simulink model "Controlled_full_wave_AC_DC_Wave_SEDC_motor_model"  (R2018a)
settings: Solver=VariableStepAuto  StartTime=0.0  StopTime=0.04  FixedStep=10e-3  MaxStep=10e-3  RelTol=1e-3
values from neighbouring files (symbols this model uses):
  B = 0.01    [AC_DC_Wave_DC_motor_parameters.m]
  J = 5    [AC_DC_Wave_DC_motor_parameters.m]
  K_phi = 1.6    [AC_DC_Wave_DC_motor_parameters.m]
  L = 0.1    [AC_DC_Wave_DC_motor_parameters.m]
  Ra = 0.5    [AC_DC_Wave_DC_motor_parameters.m]
  T_l = 10    [AC_DC_Wave_DC_motor_parameters.m]
libraries: powerlib x12, simulink x2, dspswit3 x1
settings Model: Creator=dell  LastModifiedBy=dell

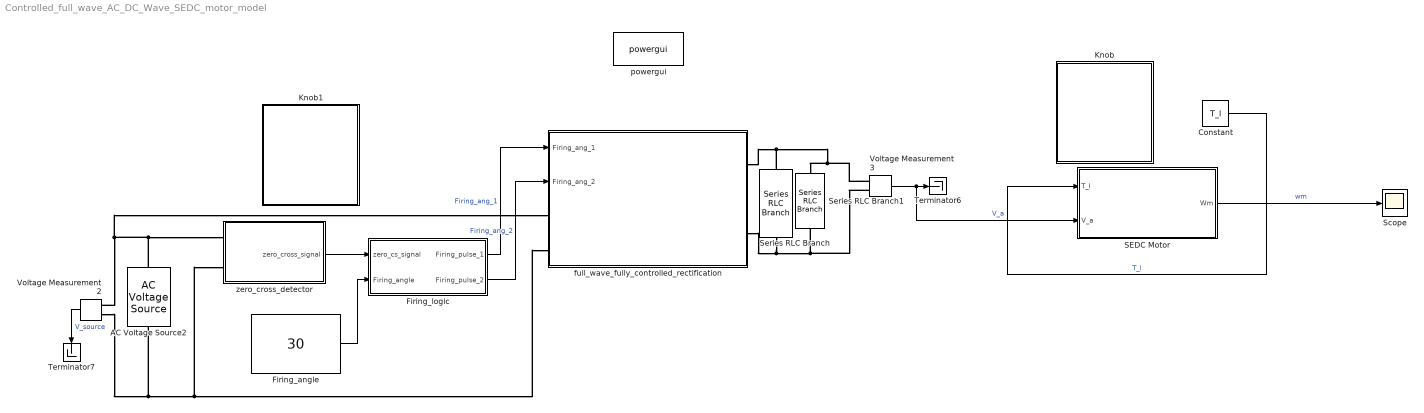
== system Controlled_full_wave_AC_DC_Wave_SEDC_motor_model ==
  AC Voltage Source2 : powerlib/Electrical Sources/AC Voltage Source  Amplitude=sqrt(2)*220  Phase=0  Frequency=50  SampleTime=0  Measurements=None  BusType=swing  Pref=10e3  Qref=0  Qmin=-inf  Qmax=+inf
  Constant : Constant  Value=T_l
  Firing_angle : Constant  Value=30
  Firing_logic : Subsystem
  Knob : Subsystem  DialogController=hmiCreateDDGDialog  IsWebBlock=on  mask(MWDashboardBlock){webBlockId=27bb38d2-9cd0-4bde-b8da-2d6c9efb7173, webBlockType=continuousknob, ShowInLibBrowser=on, ShowInitialText=on, HMISrcModelName=Controlled_full_wave_AC_DC_Wave_SEDC_motor_model}
      mask prompts: webBlockId "WebBlock Id"; webBlockType "WebBlock Type"; HMISrcModelName "Source Model"
      mask help: SimulinkHMI:dialogs:ContinuousKnobDialogDesc
      mask Help: helpview([docroot '/mapfiles/simulink.map'], 'hmi_knob')
      mask Display:
      | if strcmp(get_param(bdroot(gcb),'BlockDiagramType'), 'library')
      |     image([(matlabroot) '/toolbox/simulink/hmi/icons/ContinuousKnob.png']);
      | end
  Knob1 : Subsystem  DialogController=hmiCreateDDGDialog  IsWebBlock=on  mask(MWDashboardBlock){webBlockId=f64e203f-17e4-4edd-b46c-2720ed8f6d71, webBlockType=continuousknob, ShowInLibBrowser=on, ShowInitialText=on, HMISrcModelName=Controlled_full_wave_AC_DC_Wave_SEDC_motor_model}
      mask prompts: webBlockId "WebBlock Id"; webBlockType "WebBlock Type"; HMISrcModelName "Source Model"
      mask help: SimulinkHMI:dialogs:ContinuousKnobDialogDesc
      mask Help: helpview([docroot '/mapfiles/simulink.map'], 'hmi_knob')
      mask Display:
      | if strcmp(get_param(bdroot(gcb),'BlockDiagramType'), 'library')
      |     image([(matlabroot) '/toolbox/simulink/hmi/icons/ContinuousKnob.png']);
      | end
  SEDC Motor : Subsystem  mask{L=L, Ra=Ra, B=B, K_phi=K_phi, J=J}
      mask prompts: L "Inductance"; Ra "Resistance"; B "Damping"; K_phi "Motor Constant"; J "Inertia"
  Scope : Scope
  Series RLC Branch : powerlib/Elements/Series RLC Branch  LConnTagsString=__new0  RConnTagsString=__new0  BranchType=C  Resistance=1  Inductance=1e-3  SetiL0=off  InitialCurrent=0  Capacitance=1  Setx0=off  InitialVoltage=0  Measurements=None
  Series RLC Branch1 : powerlib/Elements/Series RLC Branch  LConnTagsString=__new0  RConnTagsString=__new0  BranchType=R  Resistance=50  Inductance=1e-3  SetiL0=off  InitialCurrent=0  Capacitance=1e-6  Setx0=off  InitialVoltage=0  Measurements=None
  Terminator6 : Terminator
  Terminator7 : Terminator
  Voltage Measurement2 : powerlib/Measurements/Voltage Measurement  PhasorSimulation=off  OutputType=Complex  PSBequivalent=0
  Voltage Measurement3 : powerlib/Measurements/Voltage Measurement  PhasorSimulation=off  OutputType=Complex  PSBequivalent=0
  full_wave_fully_controlled_rectification : Subsystem
  powergui : powerlib/powergui  Priority=1  SimulationMode=Discrete  SampleTime=50e-6  frequency=60  Iterations=50  frequencyindice=0  Pbase=100e6  ErrMax=1e-4  UnitsV=kV  UnitsW=MW  buscounter=0  FunctionMessages=off  echomessages=off  EnableUseOfTLC=off  CurrentSourceSwitches=off  DisableSnubberDevices=off  DisableRonSwitches=off  DisableVfSwitches=off  DisplayEquations=off  SolverType=Tustin/Backward Euler (TBE)  Interpol=off  ExternalGateDelay=off  methode=off  Ts=100  x0status=blocks  SPID=off  SwTol=0  HookPort=off  RestoreLinks=warning  ResistiveCurrentMeasurement=off  Frange=[0:2:500]  Ylog=off  Xlog=on  ShowGrid=off  save=off  variable=ZData  structure=0  ZoomFFT=off  StartTime=0.0  cycles=1  DisplayStyle=1  fundamental=60  FreqAxis=off  MaxFrequency=1000  frequencyindicesteady=1  RmsSteady=1  display=off
  zero_cross_detector : Subsystem
  wires:
  Constant/1 -> SEDC Motor/1(T_l)  "T_l"
  Voltage Measurement3/1 -> SEDC Motor/2(V_a), Terminator6/1  "V_a"
  SEDC Motor/1(Wm) -> Scope/1  "wm"
  Voltage Measurement2/1 -> Terminator7/1  "V_source"
  Firing_logic/1(Firing_pulse_1) -> full_wave_fully_controlled_rectification/1(Firing_ang_1)  "Firing_ang_1"
  Firing_logic/2(Firing_pulse_2) -> full_wave_fully_controlled_rectification/2(Firing_ang_2)  "Firing_ang_2"
  zero_cross_detector/1(zero_cross_signal) -> Firing_logic/1(zero_cs_signal)
  Firing_angle/1 -> Firing_logic/2(Firing_angle)
  connections:
  AC Voltage Source2/RConn1 -- full_wave_fully_controlled_rectification/LConn1 -- Voltage Measurement2/LConn1 -- zero_cross_detector/LConn1
  Voltage Measurement2/LConn2 -- AC Voltage Source2/LConn1 -- zero_cross_detector/LConn2 -- full_wave_fully_controlled_rectification/LConn2
  full_wave_fully_controlled_rectification/RConn1 -- Series RLC Branch/LConn1 -- Series RLC Branch1/LConn1 -- Voltage Measurement3/LConn1
  full_wave_fully_controlled_rectification/RConn2 -- Series RLC Branch/RConn1 -- Voltage Measurement3/LConn2 -- Series RLC Branch1/RConn1

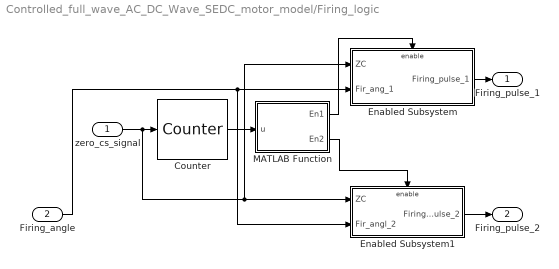
== system Controlled_full_wave_AC_DC_Wave_SEDC_motor_model/Firing_logic ==
  zero_cs_signal : Inport
  Firing_angle : Inport  Port=2
  Counter : dspswit3/Counter  Direction=Up  CountEvent=Rising edge  CounterSize=User defined  MaxCount=255  InitialCount=0  Output=Count  HitValue=32  ResetInput=off  SamplesPerFrame=1  Ts=1  CntDtype=double  HitDtype=Logical
  Enabled Subsystem : Subsystem  TreatAsAtomicUnit=on
  Enabled Subsystem1 : Subsystem  TreatAsAtomicUnit=on
  MATLAB Function : MATLAB Function  TreatAsAtomicUnit=on
  Firing_pulse_1 : Outport
  Firing_pulse_2 : Outport  Port=2
  wires:
  zero_cs_signal/1 -> Enabled Subsystem1/1(ZC), Enabled Subsystem/1(ZC), Counter/1
  Counter/1 -> MATLAB Function/1(u)
  MATLAB Function/1(En1) -> Enabled Subsystem/Enable
  MATLAB Function/2(En2) -> Enabled Subsystem1/Enable
  Firing_angle/1 -> Enabled Subsystem/2(Fir_ang_1), Enabled Subsystem1/2(Fir_angl_2)
  Enabled Subsystem/1(Firing_pulse_1) -> Firing_pulse_1/1
  Enabled Subsystem1/1(Firing_pulse_2) -> Firing_pulse_2/1

== system Controlled_full_wave_AC_DC_Wave_SEDC_motor_model/Knob ==

== system Controlled_full_wave_AC_DC_Wave_SEDC_motor_model/Knob1 ==

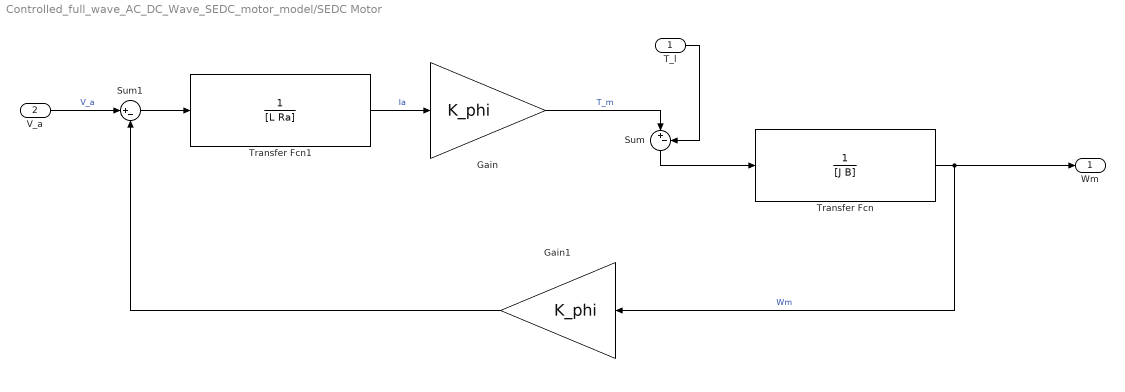
== system Controlled_full_wave_AC_DC_Wave_SEDC_motor_model/SEDC Motor ==
  T_l : Inport
  V_a : Inport  Port=2
  Gain : Gain  Gain=K_phi
  Gain1 : Gain  Gain=K_phi
  Sum : Sum  Inputs=|+-
  Sum1 : Sum  Inputs=|+-
  Transfer Fcn : TransferFcn  Denominator=[J B]
  Transfer Fcn1 : TransferFcn  Denominator=[L Ra]
  Wm : Outport
  wires:
  Gain/1 -> Sum/1  "T_m"
  Transfer Fcn1/1 -> Gain/1  "Ia"
  Transfer Fcn/1 -> Wm/1, Gain1/1  "Wm"
  Sum1/1 -> Transfer Fcn1/1
  T_l/1 -> Sum/2
  Sum/1 -> Transfer Fcn/1
  Gain1/1 -> Sum1/2
  V_a/1 -> Sum1/1  "V_a"

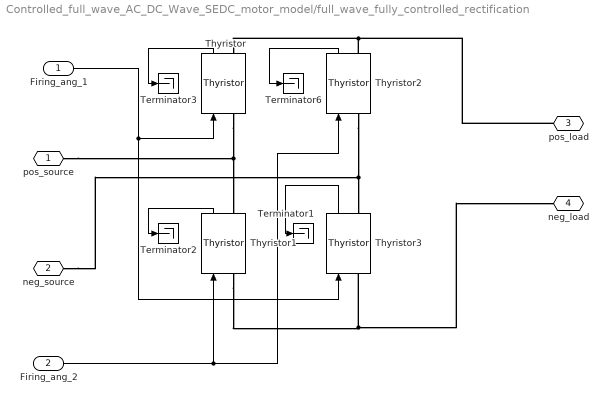
== system Controlled_full_wave_AC_DC_Wave_SEDC_motor_model/full_wave_fully_controlled_rectification ==
  Firing_ang_1 : Inport
  Firing_ang_2 : Inport  Port=2
  Terminator{1..3,6} (4 alike) : Terminator
  Thyristor{,1..3} (4 alike) : powerlib/Power Electronics/Thyristor  Ron=0.001  Lon=0  Vf=0.8  IC=0  Rs=500  Cs=250e-9  Measurements=on
  pos_source : PMIOPort  Side=Left
  neg_source : PMIOPort  Port=2  Side=Left
  pos_load : PMIOPort  Port=3  Side=Right
  "neg_load " : PMIOPort  Port=4  Side=Right
  wires:
  Firing_ang_2/1 -> Thyristor1/1, Thyristor2/1
  Thyristor3/1 -> Terminator1/1
  Thyristor2/1 -> Terminator6/1
  Firing_ang_1/1 -> Thyristor3/1, Thyristor/1
  Thyristor1/1 -> Terminator2/1
  Thyristor/1 -> Terminator3/1
  connections:
  Thyristor2/RConn1 -- pos_load/RConn1 -- Thyristor/RConn1
  Thyristor/LConn1 -- pos_source/RConn1 -- Thyristor1/RConn1
  Thyristor1/LConn1 -- "neg_load "/RConn1 -- Thyristor3/LConn1
  Thyristor2/LConn1 -- Thyristor3/RConn1 -- neg_source/RConn1

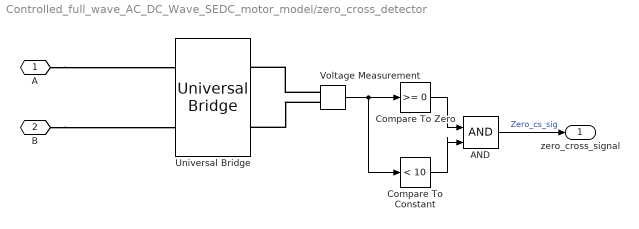
== system Controlled_full_wave_AC_DC_Wave_SEDC_motor_model/zero_cross_detector ==
  AND : Logic  IconShape=distinctive  AllPortsSameDT=off  OutDataTypeStr=boolean
  Compare To Constant : simulink/Logic and Bit Operations/Compare To Constant  relop=<  const=10  OutDataTypeStr=boolean
  Compare To Zero : simulink/Logic and Bit Operations/Compare To Zero  relop=>=  OutDataTypeStr=boolean
  Universal Bridge : powerlib/Power Electronics/Universal Bridge  Arms=2  SnubberResistance=1e5  SnubberCapacitance=inf  Device=Diodes  Ron=1e-3  Lon=0  ForwardVoltages="[  0  0  ]"  ForwardVoltage=0  GTOparameters=[ 10e-6 , 20e-6 ]  IGBTparameters=[ 1e-6 , 2e-6 ]  Measurements=None  Measurements_2=None  converterType=Rectifier
  Voltage Measurement : powerlib/Measurements/Voltage Measurement  PhasorSimulation=off  OutputType=Complex  PSBequivalent=0
  A : PMIOPort  Side=Left
  B : PMIOPort  Port=2  Side=Left
  zero_cross_signal : Outport
  wires:
  Voltage Measurement/1 -> Compare To Constant/1, Compare To Zero/1
  Compare To Zero/1 -> AND/1
  Compare To Constant/1 -> AND/2
  AND/1 -> zero_cross_signal/1  "Zero_cs_sig"
  connections:
  A/RConn1 -- Universal Bridge/LConn1
  B/RConn1 -- Universal Bridge/LConn2
  Voltage Measurement/LConn1 -- Universal Bridge/RConn1
  Voltage Measurement/LConn2 -- Universal Bridge/RConn2

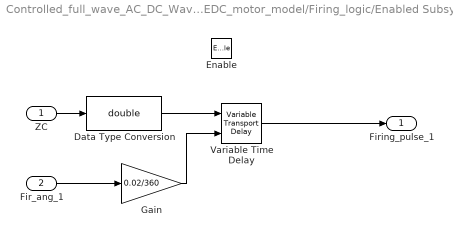
== system Controlled_full_wave_AC_DC_Wave_SEDC_motor_model/Firing_logic/Enabled Subsystem ==
  ZC : Inport
  Fir_ang_1 : Inport  Port=2
  Enable : EnablePort
  Data Type Conversion : DataTypeConversion  OutDataTypeStr=double
  Gain : Gain  Gain=0.02/360
  Variable Time Delay : VariableTransportDelay  MaximumDelay=10
  Firing_pulse_1 : Outport
  wires:
  Fir_ang_1/1 -> Gain/1
  ZC/1 -> Data Type Conversion/1
  Gain/1 -> Variable Time Delay/2
  Variable Time Delay/1 -> Firing_pulse_1/1
  Data Type Conversion/1 -> Variable Time Delay/1

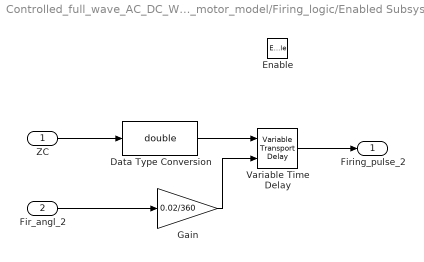
== system Controlled_full_wave_AC_DC_Wave_SEDC_motor_model/Firing_logic/Enabled Subsystem1 ==
  ZC : Inport
  Fir_angl_2 : Inport  Port=2
  Enable : EnablePort
  Data Type Conversion : DataTypeConversion  OutDataTypeStr=double
  Gain : Gain  Gain=0.02/360
  Variable Time Delay : VariableTransportDelay  MaximumDelay=10
  Firing_pulse_2 : Outport
  wires:
  Data Type Conversion/1 -> Variable Time Delay/1
  Gain/1 -> Variable Time Delay/2
  Variable Time Delay/1 -> Firing_pulse_2/1
  Fir_angl_2/1 -> Gain/1
  ZC/1 -> Data Type Conversion/1

== matlab function Controlled_full_wave_AC_DC_Wave_SEDC_motor_model/Firing_logic/MATLAB Function ==
  data: u input; En1 output; En2 output
function [En1,En2]= fcn(u)

En1 = 0;
En2 = 0;
if (mod(u,2)==0)
    En1 = 1;
    En2 = 0;
end

if(mod(u,2) == 1)
    En1 = 0;
    En2 = 1;
end
